simulink model "R3GDL_Compensador"  (R2021b)
settings: Solver=ode45  StartTime=0.0  StopTime=2  RelTol=1e-8  EnableMultiTasking=on
PreLoadFcn:
  | inicializacion
values from neighbouring files (symbols this model uses):
  Kd1 = 12/ts    (= 120)    [calculo_controlador.m]
  Kd2 = 12/ts    (= 120)    [calculo_controlador.m]
  Kd3 = 12/ts    (= 120)    [calculo_controlador.m]
  Ki1 = 0    [calculo_controlador.m]
  Ki2 = 0    [calculo_controlador.m]
  Ki3 = 0    [calculo_controlador.m]
  Kp1 = 36/ts^2    (= 3600)    [calculo_controlador.m]
  Kp2 = 36/ts^2    (= 3600)    [calculo_controlador.m]
  Kp3 = 36/ts^2    (= 3600)    [calculo_controlador.m]
  qInicial = aux(:,1)    [inicializacion.m]
  xyzFinal = xyzInicial+ [-0.15  -0.15  0.15]    [inicializacion.m]
  xyzInicial = [1.5  0.5  2.5]    [inicializacion.m]
settings Model: Creator=Manuel G. Ortega  LastModifiedBy=alvar
settings SolverCC: AlgebraicLoopSolver=TrustRegion
settings DataIOCC: SaveFormat=Array  SignalLoggingSaveFormat=ModelDataLogs  ReturnWorkspaceOutputs=off
settings OptimizationCC: BooleanDataType=off  ExpressionDepthLimit=2147483647  InitFltsAndDblsToZero=on  LifeSpan=inf
settings DebuggingCC: SaveWithParameterizedLinksMsg=none  UnderspecifiedInitializationDetection=Classic  MergeDetectMultiDrivingBlocksExec=none  SignalResolutionControl=TryResolveAllWithWarning  MultiTaskDSMMsg=warning  MultiTaskCondExecSysMsg=none  FcnCallInpInsideContextMsg=warning  StateNameClashWarn=warning  SFUnexpectedBacktrackingDiag=warning  SFNoUnconditionalDefaultTransitionDiag=warning  SFExecutionAtInitializationDiag=none  SFMachineParentedDataDiag=warning  ArithmeticOperatorsInVariantConditions=warning
settings HardwareCC: ProdBitPerPointer=32  ProdBitPerSizeT=32  ProdBitPerPtrDiffT=32  ProdLargestAtomicFloat=None  ProdIntDivRoundTo=Undefined  ProdEndianess=Unspecified  ProdWordSize=32  ProdHWDeviceType=32-bit Generic  TargetUnknown=on
settings ModelReferenceCC: PropagateSignalLabelsOutOfModel=off
settings SFSimCC: SimUseLocalCustomCode=off  CustomCodeUndefinedFunction=UseInterfaceOnly
settings RTWCC: RTWUseLocalCustomCode=off
settings CodeAppCC: StateflowObjectComments=on
settings GRTTargetCC: TargetFcnLib=ansi_tfl_tmw.mat  TargetLangStandard=C89/C90 (ANSI)  CombineOutputUpdateFcns=off  GRTInterface=on
settings ConfigComp: CovMetricSettings=dw  CovSaveCumulativeToWorkspaceVar=on  CovSaveSingleToWorkspaceVar=on  CovExternalEMLEnable=off  CovSFcnEnable=off

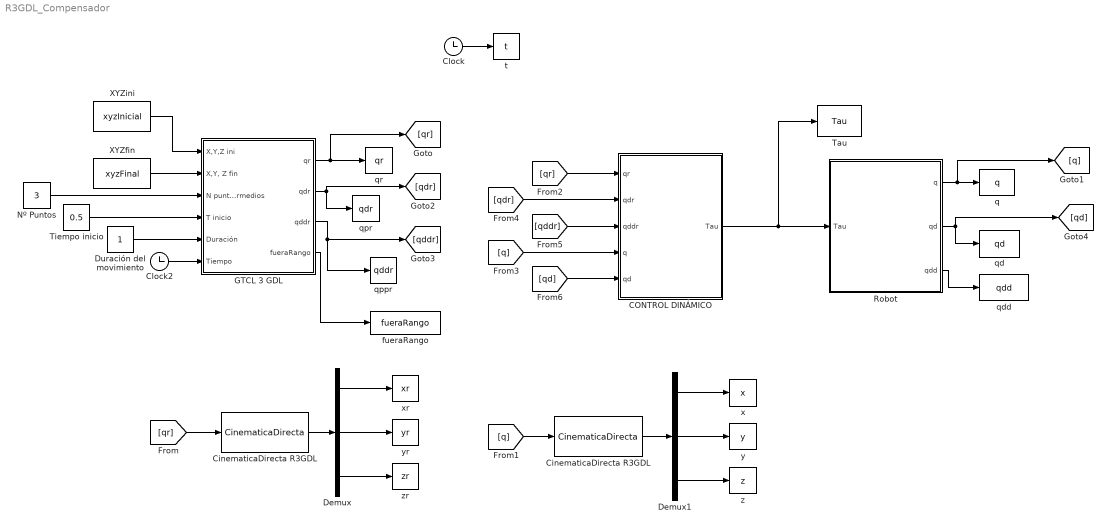
== system R3GDL_Compensador ==
  CONTROL DINÁMICO : Subsystem
  CinematicaDirecta R3GDL : MATLABFcn  MATLABFcn=CinematicaDirecta  OutputDimensions=3
  "CinematicaDirecta R3GDL " : MATLABFcn  MATLABFcn=CinematicaDirecta  OutputDimensions=3
  Clock : Clock
  Clock2 : Clock
  Demux : Demux  Outputs=3
  Demux1 : Demux  Outputs=3
  Duración del movimiento : Constant
  GTCL 3 GDL : Subsystem
  Nº Puntos : Constant  Value=3
  Robot : Subsystem
      mask Display: image('C:\Users\alvar\OneDrive\Escritorio\TRABAJO CURSO\A_Análisis_Cinemático\3\robot3gdl.jpg'); % Use "Edit Image" on toolstrip to change.
  "Tau " : ToWorkspace  VariableName=Tau  SampleTime=-1
  Tiempo inicio : Constant  Value=0.5
  XYZfin : Constant  Value=xyzFinal
  XYZini : Constant  Value=xyzInicial
  fueraRango : ToWorkspace  VariableName=fueraRango  SampleTime=-1
  q : ToWorkspace  VariableName=q  SampleTime=-1
  qd : ToWorkspace  VariableName=qd  SampleTime=-1
  qdd : ToWorkspace  VariableName=qdd  SampleTime=-1
  qppr : ToWorkspace  VariableName=qddr  SampleTime=-1
  qpr : ToWorkspace  VariableName=qdr  SampleTime=-1
  qr : ToWorkspace  VariableName=qr  SampleTime=-1
  t : ToWorkspace  VariableName=t  SampleTime=-1
  x : ToWorkspace  VariableName=x  SampleTime=-1
  xr : ToWorkspace  VariableName=xr  SampleTime=-1
  y : ToWorkspace  VariableName=y  SampleTime=-1
  yr : ToWorkspace  VariableName=yr  SampleTime=-1
  z : ToWorkspace  VariableName=z  SampleTime=-1
  zr : ToWorkspace  VariableName=zr  SampleTime=-1
  wires:
  Robot/1(q) -> [q], q/1
  Robot/2(qd) -> qd/1, [qd]
  Robot/3(qdd) -> qdd/1
  Clock/1 -> t/1
  Clock2/1 -> GTCL 3 GDL/6(Tiempo)
  Duración del movimiento/1 -> GTCL 3 GDL/5(Duración)
  Tiempo inicio/1 -> GTCL 3 GDL/4(T inicio)
  Nº Puntos/1 -> GTCL 3 GDL/3(N puntos intermedios)
  XYZfin/1 -> GTCL 3 GDL/2("X,Y, Z fin")
  XYZini/1 -> GTCL 3 GDL/1(X,Y,Z ini)
  GTCL 3 GDL/1(qr) -> [qr], qr/1
  GTCL 3 GDL/2(qdr) -> qpr/1, [qdr]
  GTCL 3 GDL/3(qddr) -> qppr/1, [qddr]
  [qr] -> CinematicaDirecta R3GDL/1
  CinematicaDirecta R3GDL/1 -> Demux/1
  Demux/1 -> xr/1
  Demux/2 -> yr/1
  Demux/3 -> zr/1
  [q] -> "CinematicaDirecta R3GDL "/1
  "CinematicaDirecta R3GDL "/1 -> Demux1/1
  Demux1/1 -> x/1
  Demux1/2 -> y/1
  Demux1/3 -> z/1
  CONTROL DINÁMICO/1(Tau) -> "Tau "/1, Robot/1(Tau)
  [qr] -> CONTROL DINÁMICO/1(qr)
  [qdr] -> CONTROL DINÁMICO/2(qdr)
  [qddr] -> CONTROL DINÁMICO/3(qddr)
  [q] -> CONTROL DINÁMICO/4(q)
  [qd] -> CONTROL DINÁMICO/5(qd)
  GTCL 3 GDL/4(fueraRango) -> fueraRango/1

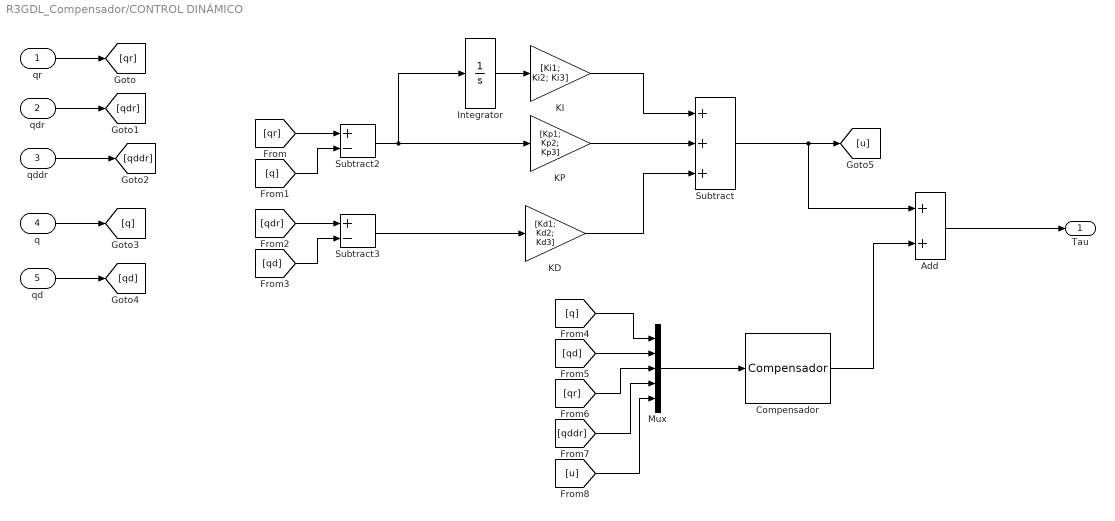
== system R3GDL_Compensador/CONTROL DINÁMICO ==
  qr : Inport
  qdr : Inport  Port=2
  qddr : Inport  Port=3
  q : Inport  Port=4
  qd : Inport  Port=5
  Add : Sum
  Compensador : MATLABFcn  MATLABFcn=Compensador  OutputDimensions=3
  Integrator : Integrator
  KD : Gain  Gain=[Kd1; Kd2; Kd3]
  KI : Gain  Gain=[Ki1; Ki2; Ki3]
  KP : Gain  Gain=[Kp1; Kp2; Kp3]
  Mux : Mux  Inputs=5
  Subtract : Sum  Inputs=+++
  Subtract2 : Sum  Inputs=+-
  Subtract3 : Sum  Inputs=+-
  Tau : Outport
  wires:
  Subtract2/1 -> Integrator/1, KP/1
  Subtract3/1 -> KD/1
  qr/1 -> [qr]
  qdr/1 -> [qdr]
  qddr/1 -> [qddr]
  q/1 -> [q]
  qd/1 -> [qd]
  [qr] -> Subtract2/1
  [q] -> Subtract2/2
  [qdr] -> Subtract3/1
  [qd] -> Subtract3/2
  KI/1 -> Subtract/1
  KP/1 -> Subtract/2
  KD/1 -> Subtract/3
  Integrator/1 -> KI/1
  Mux/1 -> Compensador/1
  [q] -> Mux/1
  [qd] -> Mux/2
  [qr] -> Mux/3
  Subtract/1 -> Add/1, [u]
  [qddr] -> Mux/4
  [u] -> Mux/5
  Compensador/1 -> Add/2
  Add/1 -> Tau/1

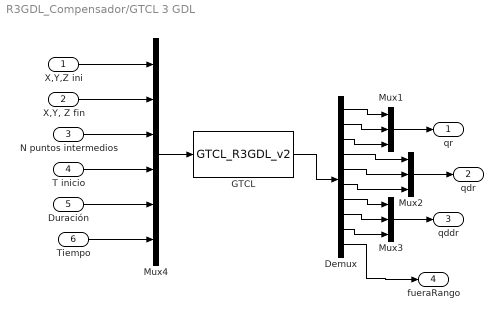
== system R3GDL_Compensador/GTCL 3 GDL ==
  X,Y,Z ini : Inport
  "X,Y, Z fin" : Inport  Port=2
  N puntos intermedios : Inport  Port=3
  T inicio : Inport  Port=4
  Duración : Inport  Port=5
  Tiempo : Inport  Port=6
  Demux : Demux  Outputs=10
  GTCL : MATLABFcn  MATLABFcn=GTCL_R3GDL_v2
  Mux1 : Mux  Inputs=3
  Mux2 : Mux  Inputs=3
  Mux3 : Mux  Inputs=3
  Mux4 : Mux  Inputs=6
  qr : Outport
  qdr : Outport  Port=2
  qddr : Outport  Port=3
  fueraRango : Outport  Port=4
  wires:
  Mux1/1 -> qr/1
  Mux4/1 -> GTCL/1
  X,Y,Z ini/1 -> Mux4/1
  "X,Y, Z fin"/1 -> Mux4/2
  N puntos intermedios/1 -> Mux4/3
  T inicio/1 -> Mux4/4
  Duración/1 -> Mux4/5
  Tiempo/1 -> Mux4/6
  GTCL/1 -> Demux/1
  Demux/1 -> Mux1/1
  Demux/2 -> Mux1/2
  Demux/3 -> Mux1/3
  Mux2/1 -> qdr/1
  Demux/4 -> Mux2/1
  Demux/5 -> Mux2/2
  Demux/6 -> Mux2/3
  Mux3/1 -> qddr/1
  Demux/7 -> Mux3/1
  Demux/8 -> Mux3/2
  Demux/9 -> Mux3/3
  Demux/10 -> fueraRango/1

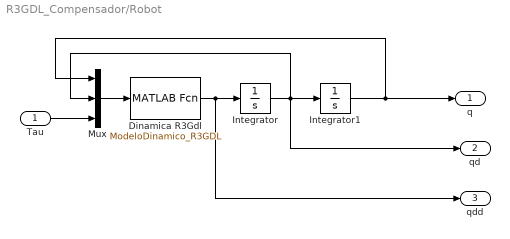
== system R3GDL_Compensador/Robot ==
  Tau : Inport
  Dinamica R3Gdl : MATLABFcn  MATLABFcn=ModeloDinamico_R3GDL  OutputDimensions=3
  Integrator : Integrator  InitialCondition=[0;0;0];
  Integrator1 : Integrator  InitialCondition=qInicial
  Mux : Mux  Inputs=3
  q : Outport
  qd : Outport  Port=2
  qdd : Outport  Port=3
  wires:
  Mux/1 -> Dinamica R3Gdl/1
  Dinamica R3Gdl/1 -> Integrator/1, qdd/1
  Integrator/1 -> Integrator1/1, qd/1, Mux/2
  Integrator1/1 -> q/1, Mux/1
  Tau/1 -> Mux/3
